simulink model "project_model"  (R2021a)
settings: Solver=FixedStepAuto  StartTime=0.0  StopTime=inf  RelTol=1e-3  EnableMultiTasking=on
undefined symbols (not defined in the file): PID
libraries: arduinolib x7, simulink x1
settings Model: SILPILModeSetting=veronly  ExtModeTrigDuration=2  Creator=asus  LastModifiedBy=asus
settings OptimizationCC: EnhancedBackFolding=on  PassReuseOutputArgsAs=Individual arguments  ZeroExternalMemoryAtStartup=off  ZeroInternalMemoryAtStartup=off  MaxStackSize=64  OptimizeBlockOrder=speed  DifferentSizesBufferReuse=on  OptimizationCustomize=off  EfficientTunableParamExpr=on
settings DebuggingCC: ParameterTunabilityLossMsg=error
settings HardwareCC: ProdBitPerInt=16  ProdBitPerPointer=16  ProdBitPerSizeT=16  ProdBitPerPtrDiffT=16  ProdLargestAtomicFloat=None  ProdWordSize=8  ProdHWDeviceType=Atmel->AVR  UseEmbeddedCoderFeatures=off
settings SFSimCC: MATLABDynamicMemAlloc=off
settings RTWCC: SystemTargetFile=ert.tlc  HardwareBoard=Arduino Uno  TemplateMakefile=ert_default_tmf  Toolchain=Arduino AVR  BuildConfiguration=Faster Runs
settings CodeAppCC: ForceParamTrailComments=on  IgnoreCustomStorageClasses=off  OperatorAnnotations=on  SimulinkDataObjDesc=on  SFDataObjDesc=on  InsertBlockDesc=on
settings ERTTargetCC: SupportContinuousTime=on  SupportNonInlinedSFcns=on  SupportVariableSizeSignals=on  ExtModeStaticAllocSize=250

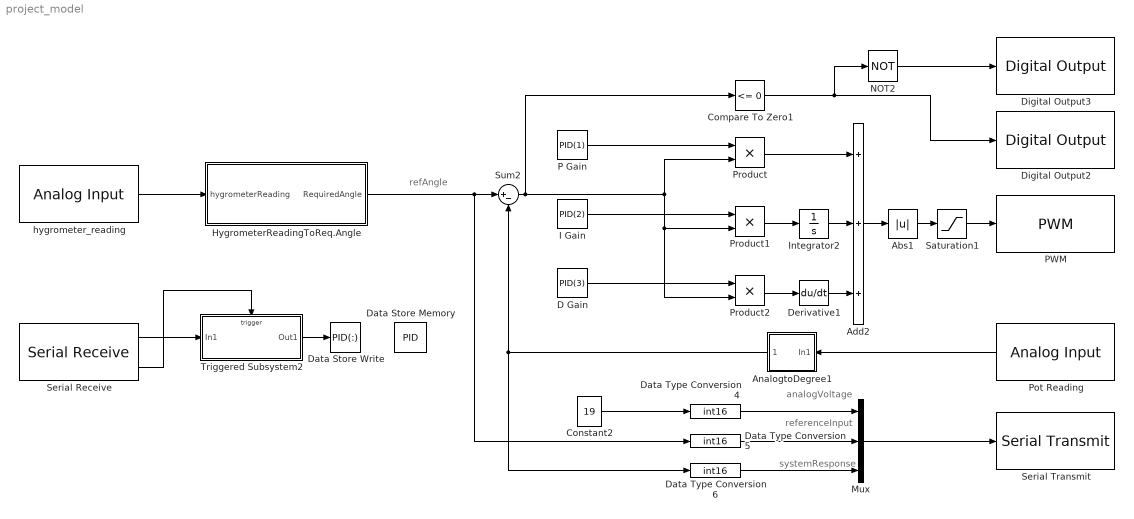
== system project_model ==
  note: refAngle
  note: analogVoltage
  note: systemResponse
  note: referenceInput
  Abs1 : Abs
  Add2 : Sum  Inputs=+++
  AnalogtoDegree1 : Subsystem
  Compare To Zero1 : simulink/Logic and Bit Operations/Compare To Zero  relop=<=  OutDataTypeStr=boolean
  Constant2 : Constant  Value=19
  D Gain : DataStoreRead  DataStoreName=PID  DataStoreElements=PID(3)  IndexOptions=Index vector (dialog)  Indices=1  OutputSizes=1
  "Data Store Memory " : DataStoreMemory  DataStoreName=PID  ReadBeforeWriteMsg=warning  WriteAfterWriteMsg=warning  WriteAfterReadMsg=warning  InitialValue=[0 0 0]  ShowAdditionalParam=off
  "Data Store Write " : DataStoreWrite  DataStoreName=PID  DataStoreElements=PID(:)  IndexOptions=Index vector (dialog)  Indices=1  OutputSizes=1
  Data Type Conversion4 : DataTypeConversion  OutDataTypeStr=int16
  Data Type Conversion5 : DataTypeConversion  OutDataTypeStr=int16
  Data Type Conversion6 : DataTypeConversion  OutDataTypeStr=int16
  Derivative1 : Derivative
  Digital Output2 : arduinolib/Digital Output  pinNumber=10  Direction=output  blockPlatform=arduino
  Digital Output3 : arduinolib/Digital Output  pinNumber=9  Direction=output  blockPlatform=arduino
  HygrometerReadingToReq.Angle : Subsystem
  I Gain : DataStoreRead  DataStoreName=PID  DataStoreElements=PID(2)  IndexOptions=Index vector (dialog)  Indices=1  OutputSizes=1
  Integrator2 : Integrator
  Mux : Mux  Inputs=3
  NOT2 : Logic  Operator=NOT  IconShape=distinctive  AllPortsSameDT=off  OutDataTypeStr=boolean
  P Gain : DataStoreRead  DataStoreName=PID  DataStoreElements=PID(1)  IndexOptions=Index vector (dialog)  Indices=1  OutputSizes=1
  "PWM " : arduinolib/PWM  pinNumber=5  frequencyType=Default  desiredFrequency=490.2  achievableFrequency=490.2
  "Pot Reading " : arduinolib/Analog Input  pinNumber=5  ReadResultsOnly=off  ConversionTriggerSource=Software  ExternalTriggerType=uint32( 0 )  OutputDataType=uint16  EnableConversionCompleteNotify=off  EnableOuputStatus=off  SampleTime=-1  blockPlatform=arduino
  Product : Product
  Product1 : Product
  Product2 : Product
  Saturation1 : Saturate  UpperLimit=80  LowerLimit=0
  "Serial Receive " : arduinolib/Serial Receive  isARMArch=off  portNumber=0  DataType=uint8  Datalength=3  SampleTime=0.1  showOutStatus=on  blockPlatform=arduino
      settings: SourceProductBaseCode=ARDUINO
  "Serial Transmit " : arduinolib/Serial Transmit  portNumber=0  sendmode=write  sendformat=Decimal  floatprecision=2  blockPlatform=arduino
  Sum2 : Sum  Inputs=|+-
  Triggered Subsystem2 : Subsystem  TreatAsAtomicUnit=on
  hygrometer_reading : arduinolib/Analog Input  pinNumber=4  ReadResultsOnly=off  ConversionTriggerSource=Software  ExternalTriggerType=uint32( 0 )  OutputDataType=uint16  EnableConversionCompleteNotify=off  EnableOuputStatus=off  SampleTime=-1  blockPlatform=arduino
  wires:
  Abs1/1 -> Saturation1/1
  Saturation1/1 -> "PWM "/1
  Integrator2/1 -> Add2/2
  "Pot Reading "/1 -> AnalogtoDegree1/1(In1)
  Sum2/1 -> Compare To Zero1/1, Product2/2, Product1/2, Product/2
  Add2/1 -> Abs1/1
  AnalogtoDegree1/1(Out1) -> Data Type Conversion6/1, Sum2/2
  NOT2/1 -> Digital Output3/1
  Compare To Zero1/1 -> NOT2/1, Digital Output2/1
  Product/1 -> Add2/1
  Mux/1 -> "Serial Transmit "/1
  Product2/1 -> Derivative1/1
  Product1/1 -> Integrator2/1
  Derivative1/1 -> Add2/3
  P Gain/1 -> Product/1
  I Gain/1 -> Product1/1
  D Gain/1 -> Product2/1
  Data Type Conversion4/1 -> Mux/1
  Data Type Conversion6/1 -> Mux/3
  Data Type Conversion5/1 -> Mux/2
  Triggered Subsystem2/1(Out1) -> "Data Store Write "/1
  "Serial Receive "/1 -> Triggered Subsystem2/1(In1)
  "Serial Receive "/2 -> Triggered Subsystem2/Trigger
  Constant2/1 -> Data Type Conversion4/1
  HygrometerReadingToReq.Angle/1(RequiredAngle) -> Data Type Conversion5/1, Sum2/1
  hygrometer_reading/1 -> HygrometerReadingToReq.Angle/1(hygrometerReading)

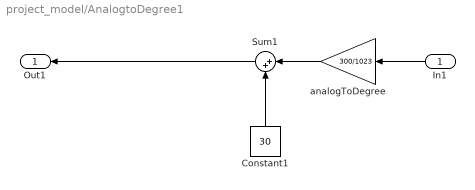
== system project_model/AnalogtoDegree1 ==
  In1 : Inport
  Constant1 : Constant  Value=30
  Sum1 : Sum  Inputs=|++
  analogToDegree : Gain  Gain=300/1023
  Out1 : Outport
  wires:
  Sum1/1 -> Out1/1
  In1/1 -> analogToDegree/1
  analogToDegree/1 -> Sum1/1
  Constant1/1 -> Sum1/2

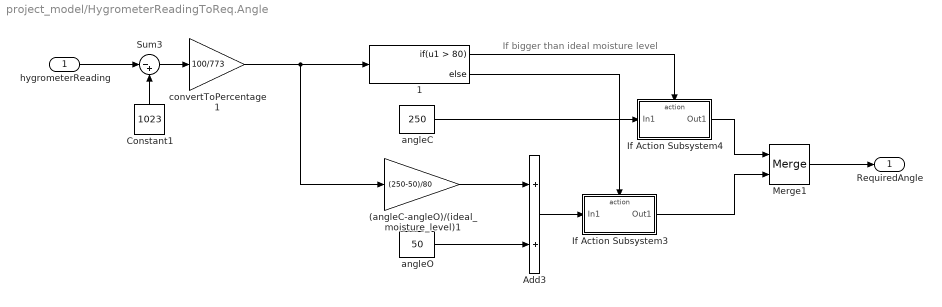
== system project_model/HygrometerReadingToReq.Angle ==
  note: If bigger than ideal moisture level
  hygrometerReading : Inport
  " 1" : If  IfExpression=u1 > 80
  (angleC-angleO)/(ideal_moisture_level)1 : Gain  Gain=(250-50)/80  OutDataTypeStr=uint8
  Add3 : Sum
  Constant1 : Constant  Value=1023
  If Action Subsystem3 : Subsystem  TreatAsAtomicUnit=on
  If Action Subsystem4 : Subsystem  TreatAsAtomicUnit=on
  Merge1 : Merge
  Sum3 : Sum  Inputs=|-+
  angleC : Constant  Value=250
  angleO : Constant  Value=50
  convertToPercentage1 : Gain  Gain=100/773  OutDataTypeStr=uint16
  RequiredAngle : Outport
  wires:
  If Action Subsystem4/1(Out1) -> Merge1/1
  convertToPercentage1/1 -> " 1"/1, (angleC-angleO)/(ideal_moisture_level)1/1
  Constant1/1 -> Sum3/2
  Sum3/1 -> convertToPercentage1/1
  (angleC-angleO)/(ideal_moisture_level)1/1 -> Add3/1
  angleC/1 -> If Action Subsystem4/1(In1)
  " 1"/2 -> If Action Subsystem3/Action
  If Action Subsystem3/1(Out1) -> Merge1/2
  " 1"/1 -> If Action Subsystem4/Action
  Add3/1 -> If Action Subsystem3/1(In1)
  angleO/1 -> Add3/2
  Merge1/1 -> RequiredAngle/1
  hygrometerReading/1 -> Sum3/1

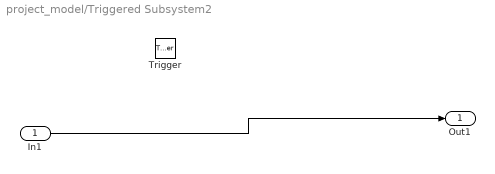
== system project_model/Triggered Subsystem2 ==
  In1 : Inport
  Trigger : TriggerPort  VariantControl=(inherit)
  Out1 : Outport
  wires:
  In1/1 -> Out1/1

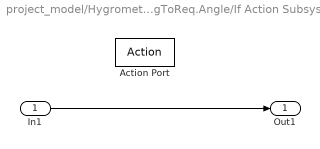
== system project_model/HygrometerReadingToReq.Angle/If Action Subsystem3 ==
  In1 : Inport
  Action Port : ActionPort  ActionPortLabel=else
  Out1 : Outport
  wires:
  In1/1 -> Out1/1

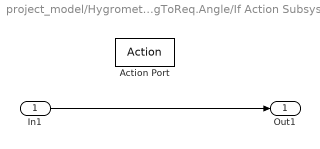
== system project_model/HygrometerReadingToReq.Angle/If Action Subsystem4 ==
  In1 : Inport
  Action Port : ActionPort  ActionPortLabel=if(u1 > 80)
  Out1 : Outport
  wires:
  In1/1 -> Out1/1
